simulink model "simulink_ex2"  (R2020a)
settings: Solver=FixedStepAuto  StartTime=0.0  StopTime=5  FixedStep=1e-3  RelTol=1e-3
settings Model: Creator=debora  LastModifiedBy=debora

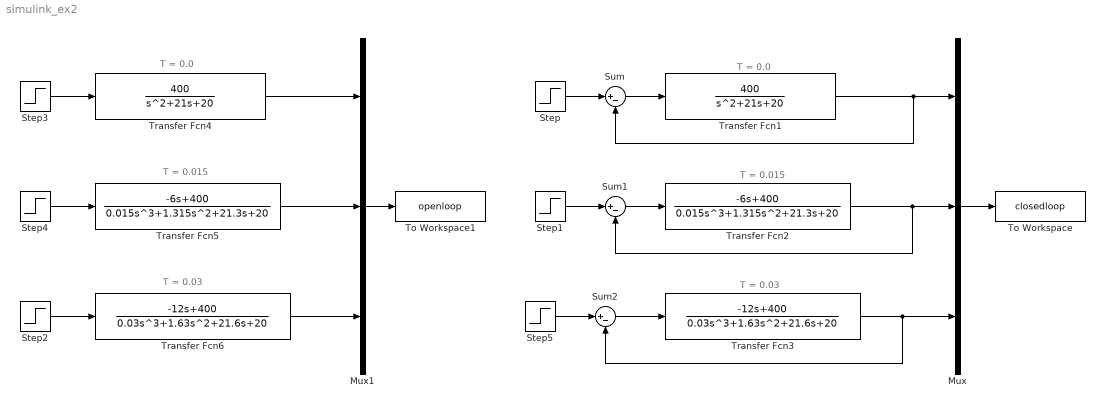
== system simulink_ex2 ==
  note: T = 0.015
  note: T = 0.0
  note: T = 0.03
  note: T = 0.0
  note: T = 0.015
  note: T = 0.03
  Mux : Mux  Inputs=3
  Mux1 : Mux  Inputs=3
  Step{,1..5} (6 alike) : Step  Time=0  SampleTime=0
  Sum : Sum  Inputs=|+-
  Sum1 : Sum  Inputs=|+-
  Sum2 : Sum  Inputs=|+-
  To Workspace : ToWorkspace  VariableName=closedloop  SaveFormat=Timeseries  SampleTime=-1
  To Workspace1 : ToWorkspace  VariableName=openloop  SaveFormat=Timeseries  SampleTime=-1
  Transfer Fcn1 : TransferFcn  Numerator=[400]  Denominator=[1 21 20]
  Transfer Fcn2 : TransferFcn  Numerator=[-6 400]  Denominator=[0.015 1.315 21.3 20]
  Transfer Fcn3 : TransferFcn  Numerator=[-12 400]  Denominator=[0.03 1.63 21.6 20]
  Transfer Fcn4 : TransferFcn  Numerator=[400]  Denominator=[1 21 20]
  Transfer Fcn5 : TransferFcn  Numerator=[-6 400]  Denominator=[0.015 1.315 21.3 20]
  Transfer Fcn6 : TransferFcn  Numerator=[-12 400]  Denominator=[0.03 1.63 21.6 20]
  wires:
  Sum/1 -> Transfer Fcn1/1
  Step/1 -> Sum/1
  Transfer Fcn1/1 -> Sum/2, Mux/1
  Step1/1 -> Sum1/1
  Transfer Fcn2/1 -> Sum1/2, Mux/2
  Sum1/1 -> Transfer Fcn2/1
  Mux/1 -> To Workspace/1
  Step3/1 -> Transfer Fcn4/1
  Step4/1 -> Transfer Fcn5/1
  Transfer Fcn4/1 -> Mux1/1
  Transfer Fcn5/1 -> Mux1/2
  Mux1/1 -> To Workspace1/1
  Step2/1 -> Transfer Fcn6/1
  Transfer Fcn6/1 -> Mux1/3
  Sum2/1 -> Transfer Fcn3/1
  Transfer Fcn3/1 -> Mux/3, Sum2/2
  Step5/1 -> Sum2/1
